simulink model "exp4_sigma"  (R2024b)
settings: Solver=ode45  StartTime=0.0  StopTime=10  MaxStep=0.01  RelTol=1e-3
settings Model: Creator=1  LastModifiedBy=1

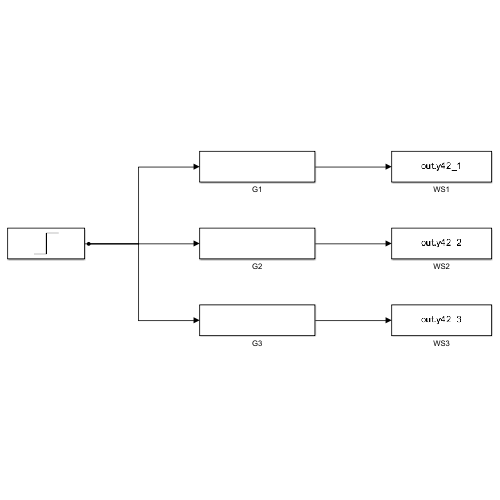
[thumbnail: Simulink's stored preview of the top-level diagram]
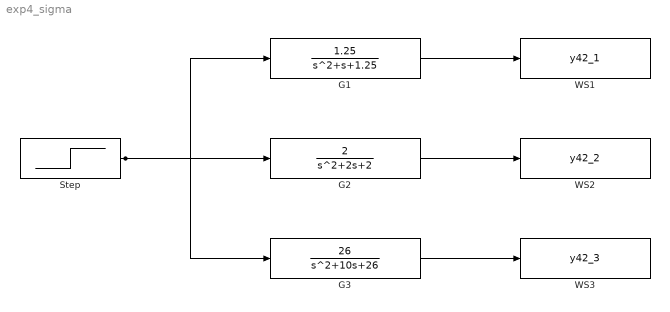
== system exp4_sigma ==
  G1 : TransferFcn  Numerator=1.25  Denominator=[1 1 1.25]
  G2 : TransferFcn  Numerator=2  Denominator=[1 2 2]
  G3 : TransferFcn  Numerator=26  Denominator=[1 10 26]
  Step : Step  Time=0  After=2  SampleTime=0
  WS1 : ToWorkspace  VariableName=y42_1  SaveFormat=Timeseries  SampleTime=-1
  WS2 : ToWorkspace  VariableName=y42_2  SaveFormat=Timeseries  SampleTime=-1
  WS3 : ToWorkspace  VariableName=y42_3  SaveFormat=Timeseries  SampleTime=-1
  wires:
  Step/1 -> G1/1, G2/1, G3/1
  G1/1 -> WS1/1
  G2/1 -> WS2/1
  G3/1 -> WS3/1
